simulink model "PV"  (R2016a)
settings: Solver=ode45  StartTime=0.0  StopTime=40  RelTol=1e-3
undefined symbols (not defined in the file): Eg0, Isc, K, ki, n, Ns, q, Rs, Rsh, Tn, Voc
libraries: simulink x3
settings Model: Creator=Sakayo Toadoum Sari  LastModifiedBy=AIMS
settings DataIOCC: LimitDataPoints=on  SaveFormat=Array
settings HardwareCC: ProdBitPerPointer=32  ProdLargestAtomicFloat=None  ProdIntDivRoundTo=Undefined  ProdEndianess=Unspecified  ProdWordSize=32  ProdHWDeviceType=32-bit Generic
settings ModelReferenceCC: PropagateSignalLabelsOutOfModel=off
settings ConfigComp: CovModelRefEnable=Off

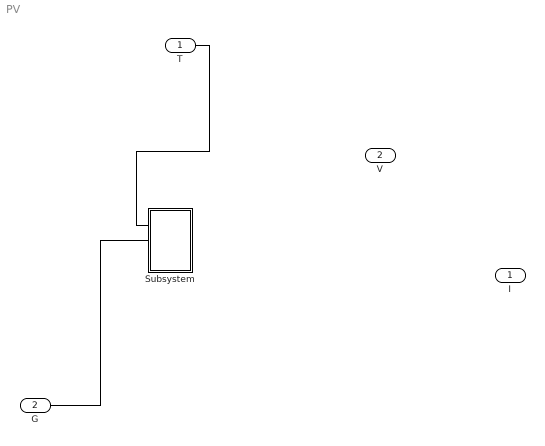
== system PV ==
  "T " : Inport
  "G " : Inport  Port=2
  Subsystem : Subsystem
  I : Outport
  V : Outport  Port=2
  wires:
  "T "/1 -> ?
  "G "/1 -> ?
  ? -> V/1
  ? -> I/1

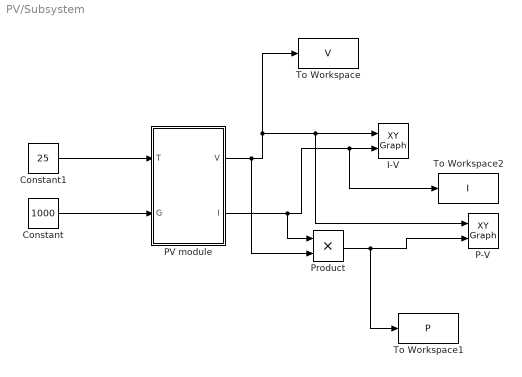
== system PV/Subsystem ==
  Constant : Constant  Value=1000
  Constant1 : Constant  Value=25
  I-V : simulink/Sinks/XY Graph  xmin=0  xmax=35  ymin=0  ymax=10  st=-1
  P-V : simulink/Sinks/XY Graph  xmin=0  xmax=35  ymin=0  ymax=210  st=-1
  PV module : Subsystem  InitFcn=|
      | ki=.0032,
      | q=1.6e-19,
      | K=1.38e-23,
      | n=1.3,
      | Eg0=1.1,
      | Rs=.221,
      | Rsh=415.405,
      | Tn=298,
      | 
      | Voc=32.9,
      | Isc=8.21,
      | Ns=54,
  Product : Product
  To Workspace : ToWorkspace  VariableName=V  SampleTime=.01
      settings: Decimation=2
  To Workspace1 : ToWorkspace  VariableName=P  SampleTime=.01
      settings: Decimation=2
  To Workspace2 : ToWorkspace  VariableName=I  SampleTime=.01
      settings: Decimation=2
  wires:
  Constant/1 -> PV module/2("G ")
  Constant1/1 -> PV module/1("T ")
  PV module/2("I ") -> Product/1, To Workspace2/1, I-V/2
  PV module/1(V) -> Product/2, To Workspace/1, P-V/1, I-V/1
  Product/1 -> To Workspace1/1, P-V/2

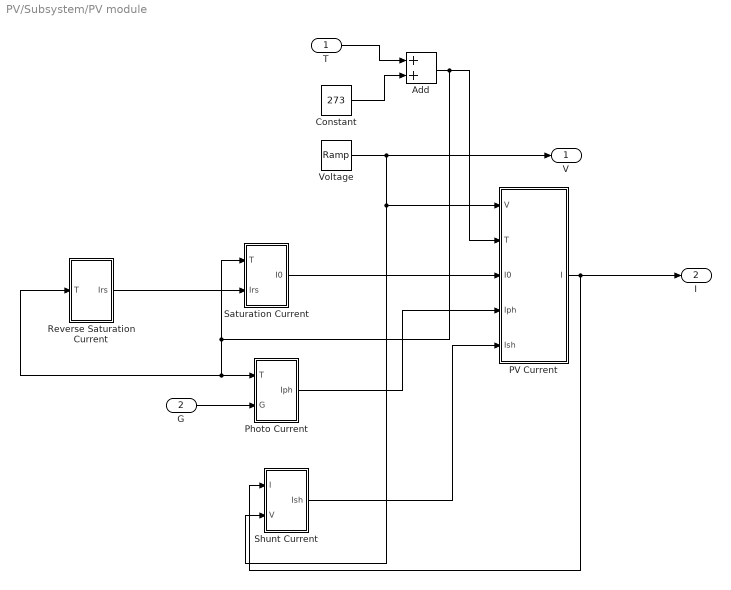
== system PV/Subsystem/PV module ==
  "T " : Inport
  "G " : Inport  Port=2
  Add : Sum
  Constant : Constant  Value=273
  "PV Current " : Subsystem
  "Photo Current " : Subsystem
  Reverse Saturation Current : Subsystem
  "Saturation Current " : Subsystem
  "Shunt Current " : Subsystem
  "Voltage " : simulink/Sources/Ramp  slope=1  start=0  X0=0
  V : Outport
  "I " : Outport  Port=2
  wires:
  "Voltage "/1 -> V/1, "Shunt Current "/2("V "), "PV Current "/1(V)
  "PV Current "/1("I ") -> "I "/1, "Shunt Current "/1(I)
  "T "/1 -> Add/1
  Reverse Saturation Current/1("Irs ") -> "Saturation Current "/2(Irs)
  "Saturation Current "/1("I0 ") -> "PV Current "/3(I0)
  Constant/1 -> Add/2
  Add/1 -> "Saturation Current "/1(T), "Photo Current "/1(T), Reverse Saturation Current/1(T), "PV Current "/2(T)
  "G "/1 -> "Photo Current "/2(G)
  "Shunt Current "/1(Ish) -> "PV Current "/5("Ish ")
  "Photo Current "/1("Iph ") -> "PV Current "/4(Iph)

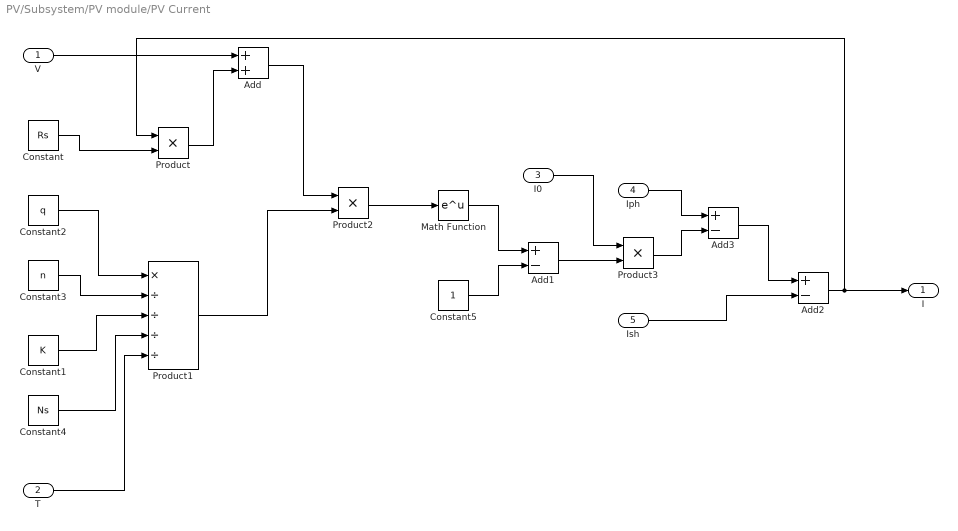
== system PV/Subsystem/PV module/PV Current  ==
  V : Inport
  T : Inport  Port=2
  I0 : Inport  Port=3
  Iph : Inport  Port=4
  "Ish " : Inport  Port=5
  Add : Sum
  Add1 : Sum  Inputs=+-
  Add2 : Sum  Inputs=+-
  Add3 : Sum  Inputs=+-
  Constant : Constant  Value=Rs
  Constant1 : Constant  Value=K
  Constant2 : Constant  Value=q
  Constant3 : Constant  Value=n
  Constant4 : Constant  Value=Ns
  Constant5 : Constant
  Math Function : Math  SaturateOnIntegerOverflow=on
  Product : Product
  Product1 : Product  Inputs=*////
  Product2 : Product
  Product3 : Product
  "I " : Outport
  wires:
  Iph/1 -> Add3/1
  Constant1/1 -> Product1/3
  Constant4/1 -> Product1/4
  Constant2/1 -> Product1/1
  Product2/1 -> Math Function/1
  Add1/1 -> Product3/2
  Math Function/1 -> Add1/1
  T/1 -> Product1/5
  Add3/1 -> Add2/1
  Product3/1 -> Add3/2
  "Ish "/1 -> Add2/2
  Product1/1 -> Product2/2
  Add/1 -> Product2/1
  V/1 -> Add/1
  Constant5/1 -> Add1/2
  Constant/1 -> Product/2
  I0/1 -> Product3/1
  Constant3/1 -> Product1/2
  Add2/1 -> "I "/1, Product/1
  Product/1 -> Add/2

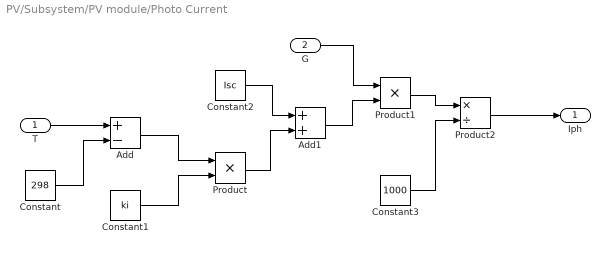
== system PV/Subsystem/PV module/Photo Current  ==
  T : Inport
  G : Inport  Port=2
  Add : Sum  Inputs=+-
  Add1 : Sum
  Constant : Constant  Value=298
  Constant1 : Constant  Value=ki
  Constant2 : Constant  Value=Isc
  Constant3 : Constant  Value=1000
  Product : Product
  Product1 : Product
  Product2 : Product  Inputs=*/
  "Iph " : Outport
  wires:
  Product/1 -> Add1/2
  Constant2/1 -> Add1/1
  Constant1/1 -> Product/2
  G/1 -> Product1/1
  Product1/1 -> Product2/1
  Product2/1 -> "Iph "/1
  T/1 -> Add/1
  Add/1 -> Product/1
  Constant/1 -> Add/2
  Add1/1 -> Product1/2
  Constant3/1 -> Product2/2

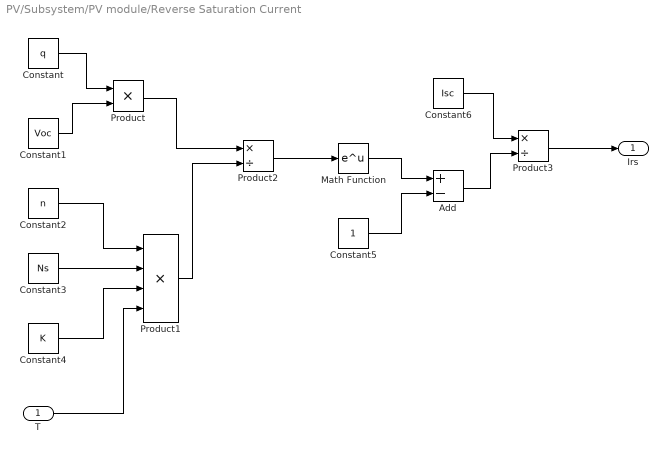
== system PV/Subsystem/PV module/Reverse Saturation Current ==
  T : Inport
  Add : Sum  Inputs=+-
  Constant : Constant  Value=q
  Constant1 : Constant  Value=Voc
  Constant2 : Constant  Value=n
  Constant3 : Constant  Value=Ns
  Constant4 : Constant  Value=K
  Constant5 : Constant
  Constant6 : Constant  Value=Isc
  Math Function : Math  SaturateOnIntegerOverflow=on
  Product : Product
  Product1 : Product  Inputs=4
  Product2 : Product  Inputs=*/
  Product3 : Product  Inputs=*/
  "Irs " : Outport
  wires:
  Product3/1 -> "Irs "/1
  Constant3/1 -> Product1/2
  Constant2/1 -> Product1/1
  Add/1 -> Product3/2
  Constant5/1 -> Add/2
  Constant/1 -> Product/1
  Product2/1 -> Math Function/1
  Constant6/1 -> Product3/1
  Math Function/1 -> Add/1
  Constant1/1 -> Product/2
  T/1 -> Product1/4
  Product1/1 -> Product2/2
  Product/1 -> Product2/1
  Constant4/1 -> Product1/3

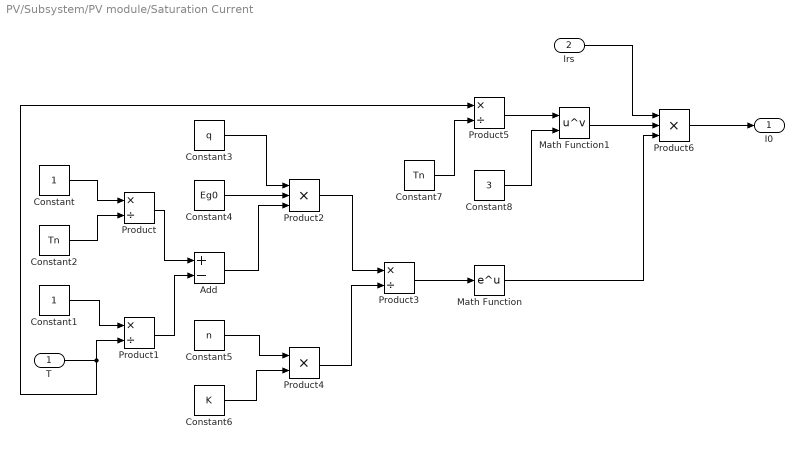
== system PV/Subsystem/PV module/Saturation Current  ==
  T : Inport
  Irs : Inport  Port=2
  Add : Sum  Inputs=+-
  Constant : Constant
  Constant1 : Constant
  Constant2 : Constant  Value=Tn
  Constant3 : Constant  Value=q
  Constant4 : Constant  Value=Eg0
  Constant5 : Constant  Value=n
  Constant6 : Constant  Value=K
  Constant7 : Constant  Value=Tn
  Constant8 : Constant  Value=3
  Math Function : Math  SaturateOnIntegerOverflow=on
  Math Function1 : Math  Operator=pow  SaturateOnIntegerOverflow=on
  Product{,1,3,5} (4 alike) : Product  Inputs=*/
  Product2 : Product  Inputs=***
  Product4 : Product  Inputs=**
  Product6 : Product  Inputs=***
  "I0 " : Outport
  wires:
  Constant6/1 -> Product4/2
  Product5/1 -> Math Function1/1
  Math Function1/1 -> Product6/2
  Math Function/1 -> Product6/3
  Irs/1 -> Product6/1
  Constant7/1 -> Product5/2
  Constant8/1 -> Math Function1/2
  Product6/1 -> "I0 "/1
  Constant/1 -> Product/1
  Constant2/1 -> Product/2
  Constant1/1 -> Product1/1
  Add/1 -> Product2/3
  Product1/1 -> Add/2
  Constant3/1 -> Product2/1
  T/1 -> Product1/2, Product5/1
  Product2/1 -> Product3/1
  Product/1 -> Add/1
  Product3/1 -> Math Function/1
  Constant5/1 -> Product4/1
  Constant4/1 -> Product2/2
  Product4/1 -> Product3/2

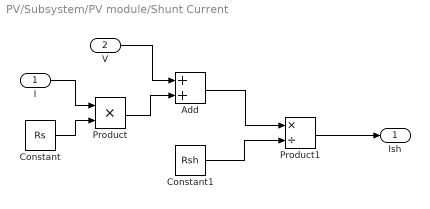
== system PV/Subsystem/PV module/Shunt Current  ==
  I : Inport
  "V " : Inport  Port=2
  Add : Sum
  Constant : Constant  Value=Rs
  Constant1 : Constant  Value=Rsh
  Product : Product
  Product1 : Product  Inputs=*/
  Ish : Outport
  wires:
  Add/1 -> Product1/1
  "V "/1 -> Add/1
  I/1 -> Product/1
  Constant/1 -> Product/2
  Constant1/1 -> Product1/2
  Product1/1 -> Ish/1
  Product/1 -> Add/2
